simulink model "Example4"  (Simulink 6.0)
settings: Solver=ode45  StartTime=0.0  StopTime=10.0  RelTol=1e-3
settings Model: LastModifiedBy=Administrator

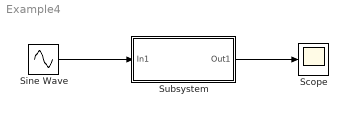
== system Example4 ==
  Scope : Scope
  Sine Wave : Sin  SampleTime=0
  Subsystem : Subsystem
  wires:
  Sine Wave/1 -> Subsystem/1(In1)
  Subsystem/1(Out1) -> Scope/1

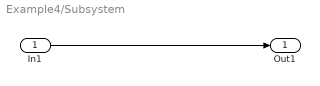
== system Example4/Subsystem ==
  In1 : Inport  Port=1  LatchInput=off
  Out1 : Outport
  wires:
  In1/1 -> Out1/1
